simulink model "hw3p2"  (R2017a)
settings: Solver=VariableStepAuto  StartTime=0.0  StopTime=10.0  RelTol=1e-3
settings Model: Creator=Soutrik  LastModifiedBy=Soutrik

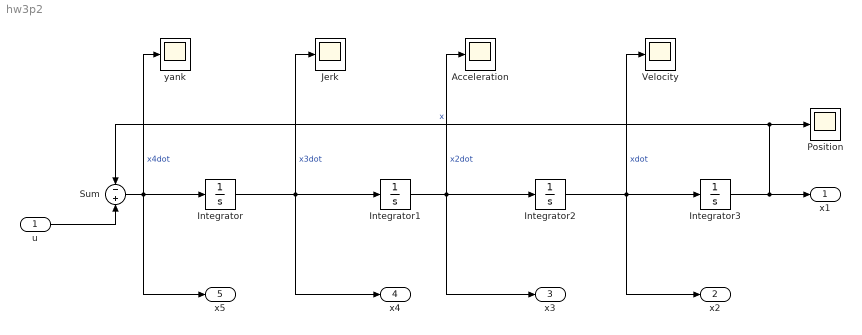
== system hw3p2 ==
  u : Inport
  Acceleration : Scope
  Integrator{,1..3} (4 alike) : Integrator
  Jerk : Scope
  Position : Scope
  Sum : Sum  Inputs=-+
  Velocity : Scope
  yank : Scope
  x1 : Outport
  x2 : Outport  Port=2
  x3 : Outport  Port=3
  x4 : Outport  Port=4
  x5 : Outport  Port=5
  wires:
  u/1 -> Sum/2
  Integrator3/1 -> x1/1, Position/1, Sum/1  "x"
  Integrator1/1 -> Integrator2/1, Acceleration/1, x3/1  "x2dot"
  Integrator/1 -> Integrator1/1, Jerk/1, x4/1  "x3dot"
  Sum/1 -> Integrator/1, yank/1, x5/1  "x4dot"
  Integrator2/1 -> Integrator3/1, Velocity/1, x2/1  "xdot"
